simulink model "MPC_RealCar_MatlabSys"  (R2023a)
settings: Solver=FixedStepAuto  StartTime=0.0  StopTime=60  FixedStep=dt  RelTol=1e-3
InitFcn:
  | Casadi_MatSys_SimulationSetup
values from neighbouring files (symbols this model uses):
  A_mat = dsys.A    [Casadi_MatSys_SimulationSetup.m]
  B_mat = dsys.B    [Casadi_MatSys_SimulationSetup.m]
  C_mat = dsys.C    [Casadi_MatSys_SimulationSetup.m]
  D_mat = 0    [Casadi_MatSys_SimulationSetup.m]
  R = 0.01*eye(1,1)    [Casadi_MatSys_SimulationSetup.m]
  r_wheel = 0.0350    (= 0.035)    [Casadi_MatSys_SimulationSetup.m]
libraries: simulink x2, realtime_pacer_lib x1
settings Model: Creator=Christian  LastModifiedBy=chris

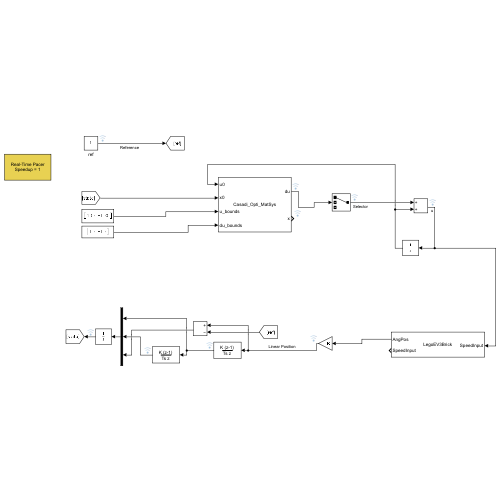
[thumbnail: Simulink's stored preview of the top-level diagram]
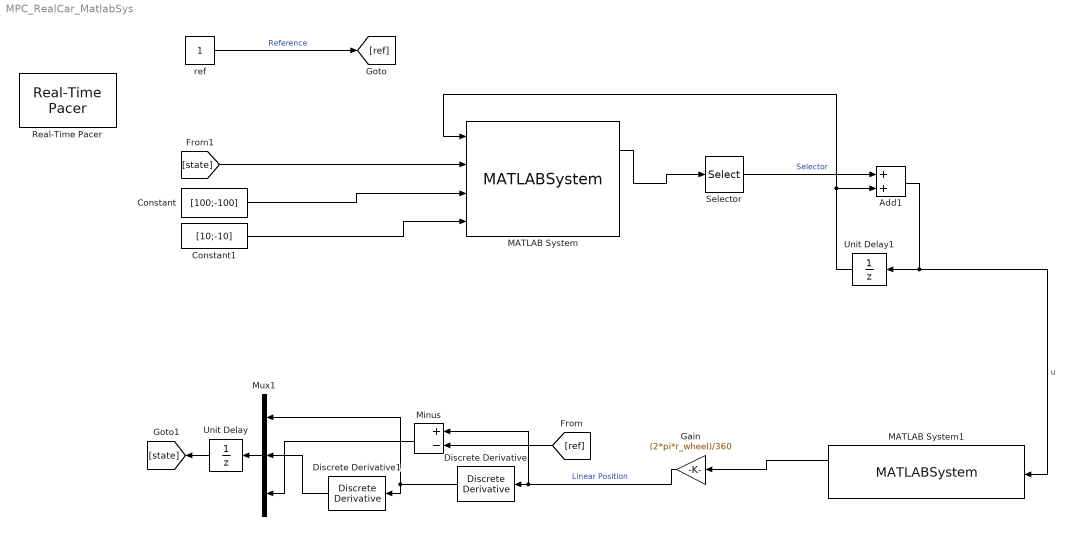
== system MPC_RealCar_MatlabSys ==
  Add1 : Sum
  Constant : Constant  Value=[100;-100]
  Constant1 : Constant  Value=[10;-10]
  Discrete Derivative : simulink/Discrete/Discrete Derivative  gainval=1.0  ICPrevScaledInput=0.0  OutMin=[]  OutMax=[]  OutDataType=fixdt(1, 16)  OutScaling=2^-10  DoSatur=off
  Discrete Derivative1 : simulink/Discrete/Discrete Derivative  gainval=1.0  ICPrevScaledInput=0.0  OutMin=[]  OutMax=[]  OutDataType=fixdt(1, 16)  OutScaling=2^-10  DoSatur=off
  Gain : Gain  Gain=(2*pi*r_wheel)/360
  MATLAB System : MATLABSystem  System=Casadi_Opti_MatSys  A=A_mat  B=B_mat  C=C_mat  D=D_mat  dt=1  N=3  Q=Q  R=R  E=E  SimulateUsing=Interpreted execution
      mask Type: Casadi_Opti_MatSys
      mask Display:
      | disp('Casadi_Opti_MatSys');
      | port_label('input',1,'u0');
      | port_label('input',2,'x0');
      | port_label('input',3,'u_bounds');
      | port_label('input',4,'du_bounds');
      | port_label('output',1,'du');
      | port_label('output',2,'x');
  MATLAB System1 : MATLABSystem  System=LegoEV3Brick  address=192.168.1.70  motorport=A  id=0016534cde97  retry_attempts=5  SimulateUsing=Interpreted execution
      mask Type: LegoEV3Brick
      mask Display:
      | disp('LegoEV3Brick');
      | port_label('input',1,'SpeedInput');
      | port_label('output',1,'AngPos');
      | port_label('output',2,'SpeedInput');
  Minus : Sum  Inputs=+-
  Mux1 : Mux  Inputs=3
  Real-Time Pacer : realtime_pacer_lib/Real-Time Pacer  simTimePerRealTime=1
      settings: SourceProductName=Real-Time Pacer
  Selector : Selector  InputPortWidth=3  IndexOptions=Index vector (dialog)  Indices=[1]  OutputSizes=1
  Unit Delay : UnitDelay  SampleTime=-1  HasFrameUpgradeWarning=on
  Unit Delay1 : UnitDelay  SampleTime=-1  HasFrameUpgradeWarning=on
  ref : Constant
  wires:
  Unit Delay/1 -> [state]
  Mux1/1 -> Unit Delay/1
  Gain/1 -> Minus/1, Discrete Derivative/1  "Linear Position"
  Discrete Derivative/1 -> Discrete Derivative1/1, Mux1/1
  MATLAB System/1 -> Selector/1
  Add1/1 -> MATLAB System1/1, Unit Delay1/1  "u"
  Unit Delay1/1 -> Add1/2, MATLAB System/1
  [state] -> MATLAB System/2
  Minus/1 -> Mux1/3
  Constant1/1 -> MATLAB System/4
  Constant/1 -> MATLAB System/3
  ref/1 -> [ref]  "Reference"
  Selector/1 -> Add1/1  "Selector"
  Discrete Derivative1/1 -> Mux1/2
  [ref] -> Minus/2
  MATLAB System1/1 -> Gain/1
